simulink model "model_15"  (R2022b)
settings: Solver=VariableStepAuto  StartTime=0.0  StopTime=1500  FixedStep=1e-3  RelTol=1e-3  EnableMultiTasking=on
StopFcn:
  | ee_addSimlogTimeStamp(bdroot)
libraries: fl_lib x74, nesl_utility x53, ee_lib x22, spsRMSLib x22, eePowerMeasurement x11
(part 2 of 2)

== matlab function model_15/MATLAB Function1 ==
  data: time input; y output; ws input
function y = fcn(time,ws)
    if time == 0
        y = 0;
    elseif floor(time) == time
        y = ws;
    else
        if floor(time) ~= 0
            y = ws;
        else
            y = 0;
        end
    end
end

== matlab function model_15/MATLAB Function15 ==
  data: time input; y output; ws input
function y = fcn(time,ws)
    if time == 0
        y = 0;
    elseif floor(time) == time
        y = ws;
    else
        if floor(time) ~= 0
            y = ws;
        else
            y = 0;
        end
    end
end

== matlab function model_15/MATLAB Function16 ==
  data: time input; y output; ws input
function y = fcn(time,ws)
    if time == 0
        y = 0;
    elseif floor(time) == time
        y = ws;
    else
        if floor(time) ~= 0
            y = ws;
        else
            y = 0;
        end
    end    
end

== matlab function model_15/MATLAB Function8 ==
  data: time input; y output; ws input
function y = fcn(time,ws)
    if time == 0
        y = 0;
    elseif floor(time) == time
        y = ws;
    else
        if floor(time) ~= 0
            y = ws;
        else
            y = 0;
        end
    end
end

== matlab function model_15/MATLAB Function9 ==
  data: time input; y output; ws input
function y = fcn(time,ws)
    if time == 0
        y = 0;
    elseif floor(time) == time
        y = ws;
    else
        if floor(time) ~= 0
            y = ws;
        else
            y = 0;
        end
    end    
end

== matlab function model_15/MATLAB Function17 ==
  data: time input; y output; ws input
function y = fcn(time,ws)
    if time == 0
        y = 0;
    elseif floor(time) == time
        y = ws;
    else
        if floor(time) ~= 0
            y = ws;
        else
            y = 0;
        end
    end
end

== matlab function model_15/MATLAB Function18 ==
  data: time input; y output; ws input
function y = fcn(time,ws)
    if time == 0
        y = 0;
    elseif floor(time) == time
        y = ws;
    else
        if floor(time) ~= 0
            y = ws;
        else
            y = 0;
        end
    end    
end

== matlab function model_15/MATLAB Function19 ==
  data: time input; y output; ws input
function y = fcn(time,ws)
    if time == 0
        y = 0;
    elseif floor(time) == time
        y = ws;
    else
        if floor(time) ~= 0
            y = ws;
        else
            y = 0;
        end
    end
end

== matlab function model_15/MATLAB Function20 ==
  data: time input; y output; ws input
function y = fcn(time,ws)
    if time == 0
        y = 0;
    elseif floor(time) == time
        y = ws;
    else
        if floor(time) ~= 0
            y = ws;
        else
            y = 0;
        end
    end    
end

== matlab function model_15/MATLAB Function21 ==
  data: time input; y output; ws input
function y = fcn(time,ws)
    if time == 0
        y = 0;
    elseif floor(time) == time
        y = ws;
    else
        if floor(time) ~= 0
            y = ws;
        else
            y = 0;
        end
    end
end

== matlab function model_15/MATLAB Function22 ==
  data: time input; y output; ws input
function y = fcn(time,ws)
    if time == 0
        y = 0;
    elseif floor(time) == time
        y = ws;
    else
        if floor(time) ~= 0
            y = ws;
        else
            y = 0;
        end
    end
end

== matlab function model_15/MATLAB Function2 ==
  data: time input; y output; ws input
function y = fcn(time,ws)
    if time == 0
        y = 0;
    elseif floor(time) == time
        y = ws;
    else
        if floor(time) ~= 0
            y = ws;
        else
            y = 0;
        end
    end
end

== matlab function model_15/MATLAB Function23 ==
  data: time input; y output; ws input
function y = fcn(time,ws)
    if time == 0
        y = 0;
    elseif floor(time) == time
        y = ws;
    else
        if floor(time) ~= 0
            y = ws;
        else
            y = 0;
        end
    end
end

== matlab function model_15/MATLAB Function24 ==
  data: time input; y output; ws input
function y = fcn(time,ws)
    if time == 0
        y = 0;
    elseif floor(time) == time
        y = ws;
    else
        if floor(time) ~= 0
            y = ws;
        else
            y = 0;
        end
    end
end

== matlab function model_15/MATLAB Function25 ==
  data: time input; y output; ws input
function y = fcn(time,ws)
    if time == 0
        y = 0;
    elseif floor(time) == time
        y = ws;
    else
        if floor(time) ~= 0
            y = ws;
        else
            y = 0;
        end
    end
end

== matlab function model_15/MATLAB Function26 ==
  data: time input; y output; ws input
function y = fcn(time,ws)
    if time == 0
        y = 0;
    elseif floor(time) == time
        y = ws;
    else
        if floor(time) ~= 0
            y = ws;
        else
            y = 0;
        end
    end
end

== matlab function model_15/MATLAB Function27 ==
  data: time input; y output; ws input
function y = fcn(time,ws)
    if time == 0
        y = 0;
    elseif floor(time) == time
        y = ws;
    else
        if floor(time) ~= 0
            y = ws;
        else
            y = 0;
        end
    end
end

== matlab function model_15/MATLAB Function28 ==
  data: time input; y output; ws input
function y = fcn(time,ws)
    if time == 0
        y = 0;
    elseif floor(time) == time
        y = ws;
    else
        if floor(time) ~= 0
            y = ws;
        else
            y = 0;
        end
    end
end

== matlab function model_15/MATLAB Function29 ==
  data: time input; y output; ws input
function y = fcn(time,ws)
    if time == 0
        y = 0;
    elseif floor(time) == time
        y = ws;
    else
        if floor(time) ~= 0
            y = ws;
        else
            y = 0;
        end
    end
end

== matlab function model_15/MATLAB Function30 ==
  data: time input; y output; ws input
function y = fcn(time,ws)
    if time == 0
        y = 0;
    elseif floor(time) == time
        y = ws;
    else
        if floor(time) ~= 0
            y = ws;
        else
            y = 0;
        end
    end
end

== matlab function model_15/MATLAB Function3 ==
  data: time input; y output; ws input
function y = fcn(time,ws)
    if time == 0
        y = 0;
    elseif floor(time) == time
        y = ws;
    else
        if floor(time) ~= 0
            y = ws;
        else
            y = 0;
        end
    end    
end

== matlab function model_15/MATLAB Function4 ==
  data: time input; y output; ws input
function y = fcn(time,ws)
    if time == 0
        y = 0;
    elseif floor(time) == time
        y = ws;
    else
        if floor(time) ~= 0
            y = ws;
        else
            y = 0;
        end
    end
end

== matlab function model_15/MATLAB Function5 ==
  data: time input; y output; ws input
function y = fcn(time,ws)
    if time == 0
        y = 0;
    elseif floor(time) == time
        y = ws;
    else
        if floor(time) ~= 0
            y = ws;
        else
            y = 0;
        end
    end    
end

== matlab function model_15/MATLAB Function6 ==
  data: time input; y output; ws input
function y = fcn(time,ws)
    if time == 0
        y = 0;
    elseif floor(time) == time
        y = ws;
    else
        if floor(time) ~= 0
            y = ws;
        else
            y = 0;
        end
    end
end

== matlab function model_15/MATLAB Function7 ==
  data: time input; y output; ws input
function y = fcn(time,ws)
    if time == 0
        y = 0;
    elseif floor(time) == time
        y = ws;
    else
        if floor(time) ~= 0
            y = ws;
        else
            y = 0;
        end
    end    
end

== matlab function model_15/MATLAB Function10 ==
  data: time input; y output; ws input
function y = fcn(time,ws)
    if time == 0
        y = 0;
    elseif floor(time) == time
        y = ws;
    else
        if floor(time) ~= 0
            y = ws;
        else
            y = 0;
        end
    end
end

== matlab function model_15/MATLAB Function12 ==
  data: time input; y output; ws input
function y = fcn(time,ws)
    if time == 0
        y = 0;
    elseif floor(time) == time
        y = ws;
    else
        if floor(time) ~= 0
            y = ws;
        else
            y = 0;
        end
    end    
end

== matlab function model_15/MATLAB Function13 ==
  data: time input; y output; ws input
function y = fcn(time,ws)
    if time == 0
        y = 0;
    elseif floor(time) == time
        y = ws;
    else
        if floor(time) ~= 0
            y = ws;
        else
            y = 0;
        end
    end
end

== matlab function model_15/MATLAB Function14 ==
  data: time input; y output; ws input
function y = fcn(time,ws)
    if time == 0
        y = 0;
    elseif floor(time) == time
        y = ws;
    else
        if floor(time) ~= 0
            y = ws;
        else
            y = 0;
        end
    end    
end

== matlab function model_15/MATLAB Function11 ==
  data: time input; y output; ws input
function y = fcn(time,ws)
    if time == 0
        y = 0;
    elseif floor(time) == time
        y = ws;
    else
        if floor(time) ~= 0
            y = ws;
        else
            y = 0;
        end
    end    
end
